simulink model "PID0"  (R2020b)
settings: Solver=VariableStepAuto  StartTime=0.0  StopTime=10.0  RelTol=1e-3
settings Model: Creator=MY lenovo  LastModifiedBy=MY lenovo
settings DataIOCC: SaveOutput=off  SaveTime=off

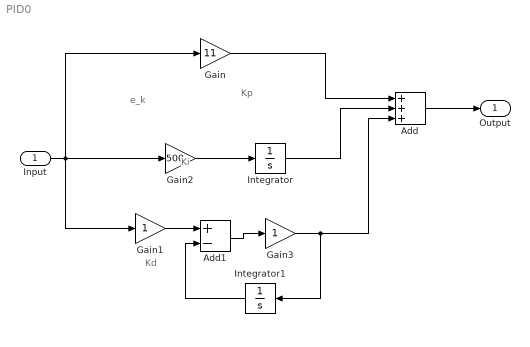
== system PID0 ==
  note: Kd
  note: Kp
  note: e_k
  note: Ki
  Input : Inport  OutDataTypeStr=double  PortDimensions=1  SampleTime=0
  Add : Sum  Inputs=+++
  Add1 : Sum  Inputs=+-
  Gain : Gain  Gain=11
  Gain1 : Gain
  Gain2 : Gain  Gain=500
  Gain3 : Gain
  Integrator : Integrator
  Integrator1 : Integrator
  Output : Outport  OutDataTypeStr=double  PortDimensions=1  SampleTime=0
  wires:
  Gain2/1 -> Integrator/1
  Integrator/1 -> Add/2
  Gain/1 -> Add/1
  Add/1 -> Output/1
  Input/1 -> Gain2/1, Gain1/1, Gain/1
  Gain1/1 -> Add1/1
  Add1/1 -> Gain3/1
  Gain3/1 -> Add/3, Integrator1/1
  Integrator1/1 -> Add1/2
